simulink model "MBD_WEEK2_QN2"  (R2020b)
settings: Solver=VariableStepAuto  StartTime=0.0  StopTime=10.0  RelTol=1e-3
values from neighbouring files (symbols this model uses):
  be = 2.0    [Variable_data.sldd]
  bv = 1.0    [Variable_data.sldd]
  Ie = 1.0    [Variable_data.sldd]
  Iv = 5.0    [Variable_data.sldd]
settings Model: Creator=dell  LastModifiedBy=dell

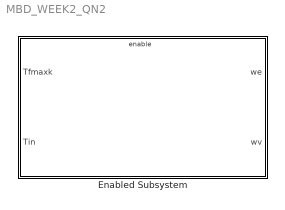
== system MBD_WEEK2_QN2 ==
  Enabled Subsystem : Subsystem  TreatAsAtomicUnit=on

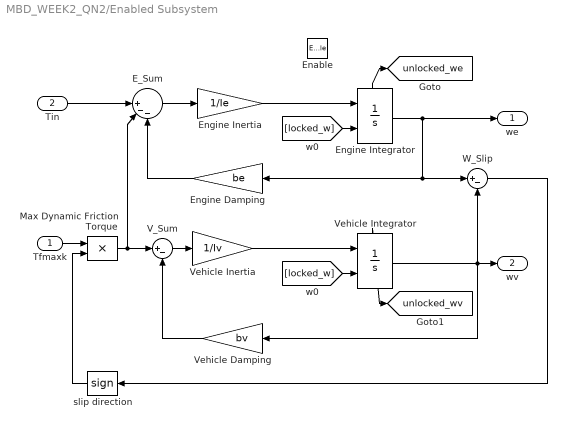
== system MBD_WEEK2_QN2/Enabled Subsystem ==
  Tfmaxk : Inport
  Tin : Inport  Port=2
  Enable : EnablePort
  E_Sum : Sum  Inputs=||+--  InputSameDT=on  SaturateOnIntegerOverflow=on  OutDataTypeStr=Inherit: Same as first input
  Engine Damping : Gain  Gain=be  SaturateOnIntegerOverflow=on  OutDataTypeStr=Inherit: Same as input  ParamDataTypeStr=Inherit: Same as input
  Engine Inertia : Gain  Gain=1/Ie  SaturateOnIntegerOverflow=on  OutDataTypeStr=Inherit: Same as input  ParamDataTypeStr=Inherit: Same as input
  Engine Integrator : Integrator  InitialConditionSource=external  ShowStatePort=on
  Max Dynamic Friction Torque : Product  InputSameDT=on  RndMeth=Zero  SaturateOnIntegerOverflow=on  OutDataTypeStr=Inherit: Same as first input
  V_Sum : Sum  Inputs=|+-  InputSameDT=on  SaturateOnIntegerOverflow=on  OutDataTypeStr=Inherit: Same as first input
  Vehicle Damping : Gain  Gain=bv  SaturateOnIntegerOverflow=on  OutDataTypeStr=Inherit: Same as input  ParamDataTypeStr=Inherit: Same as input
  Vehicle Inertia : Gain  Gain=1/Iv  SaturateOnIntegerOverflow=on  OutDataTypeStr=Inherit: Same as input  ParamDataTypeStr=Inherit: Same as input
  Vehicle Integrator : Integrator  InitialConditionSource=external  ShowStatePort=on
  W_Slip : Sum  Inputs=|+-  InputSameDT=on  SaturateOnIntegerOverflow=on  OutDataTypeStr=Inherit: Same as first input
  slip direction : Signum
  we : Outport  InitialOutput=0  VectorParamsAs1DForOutWhenUnconnected=off
  wv : Outport  Port=2  InitialOutput=0  VectorParamsAs1DForOutWhenUnconnected=off
  tag scope: unlocked_we=global, unlocked_wv=global
  wires:
  Engine Inertia/1 -> Engine Integrator/1
  E_Sum/1 -> Engine Inertia/1
  Engine Damping/1 -> E_Sum/3
  Engine Integrator/State -> [unlocked_we]
  W_Slip/1 -> slip direction/1
  slip direction/1 -> Max Dynamic Friction Torque/2
  Max Dynamic Friction Torque/1 -> V_Sum/1, E_Sum/2
  Vehicle Damping/1 -> V_Sum/2
  Tfmaxk/1 -> Max Dynamic Friction Torque/1
  Vehicle Inertia/1 -> Vehicle Integrator/1
  Vehicle Integrator/1 -> wv/1, W_Slip/2, Vehicle Damping/1
  [locked_w] -> Vehicle Integrator/2
  V_Sum/1 -> Vehicle Inertia/1
  [locked_w] -> Engine Integrator/2
  Vehicle Integrator/State -> [unlocked_wv]
  Engine Integrator/1 -> we/1, Engine Damping/1, W_Slip/1
  Tin/1 -> E_Sum/1
